simulink model "AEB_MODEL_F"  (R2022b)
settings: Solver=VariableStepAuto  StartTime=0.0  StopTime=10.0  RelTol=1e-3
model workspace (MAT data in the model file):
  DISTANCE = 100
  MASS_OF_THE_VEHICLE = 1500
  MIN_THRESHOLD_FOR_TTCmin = 0.7
  SPEED_OF_THE_EGO_VEHICLE = 80
  SPEED_OF_THE_LEADING_VEHICLE = 0
  TTC_EMERGE = 2
  Var = 0
libraries: simulink x37, spsOnDelayLib x1
(part 1 of 2)
Description:
  | VERSION 1.1
  | Done up to Brake pedal force calculation.
  | VERSION 1.2
  | Braking force applied from brake pedal force have been calculated.
  | VERSION 1.3
  | Calculating the required braking deceleration and setting the reaction time and following conditions.
  | VERSION 1.4
  | Both braking deceleration have been compared within the reaction time.
  | VERSION 1.5
  | logic gates are included to enable AEB system.
  | VERSION 1.6
  | Including some of the diagnostic check\fault and warning and condition for input range to enable AEB system through logic gate.
  | VERSION 1.7
  | Speed conversion kmph to m/s, distance to avoid collision have been calculated.
  | VERSION 1.8
  | Modelling condition for time phase partial braking.
  | VERSION 1.9
  | Modelled the condition for sudden action to apply full brake.
  | VERSION 1.10
  | Modelling the  for condition for TTCmin and TTCemerge.
  | VERSION 1.11
  | Modelling the minimum thershold for TTCmin and correcting the TTCemerge for full brake according to this TTCmin.
  | VERSION 1.12
  | Modelling the condition when to enable the full brake.
  | VERSION 1.13
  | modelled and checked the input for partial brake is correct when TTCmin have sufficient time.
  | VERSION 1.14
  | Modelling the partial brake in closed loop and limiting the braking decceleration with switch block.
  | VERSION 1.15
  | Correcting some errors by using switches and logic gates.
  | VERSION 1.16
  | Calculating the partial brake output is appropriate or not.
  | VERSION 1.17
  | Modelling the full brake in closed loop and limiting the braking decceleration with switch block.
  | VERSION 1.18
  | Recorrecting the errors occurred.
  | VERSION 1.19
  | Modelling the input condition for full brake and sudden action.
  | VERSION 1.20
  | Calculating the distance travelled after braking.
  | VERSION 1.21
  | Modelling the condition for AEB OFF at speed of ego and leading vehicle become equal.
  | VERSION 1.22
  | In output block switch is created to result the corresponding output finally.
  | VERSION 1.23
  | Indication were included for AEB status, partial brake, full brake, forward collision warning, manual mode, fault and warning.
  | VERSION 1.24
  | Updating the signal name, creating the subsystem for each calculations, proper routing line, proper naming.
  | VERSION 1.25
  | Removing the unwanted display.
  | VERSION 1.26
  | Correcting the error occurred. were the speed of ego and leading vehicle became zero AEB OFF at partial brake itself; while system is at full brake, so logic gate and switch block is included to overcome this error.
settings Model: Creator=Lenovo  LastModifiedBy=Lenovo

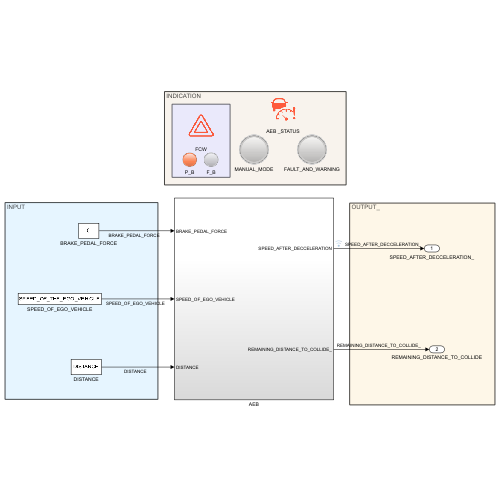
[thumbnail: Simulink's stored preview of the top-level diagram]
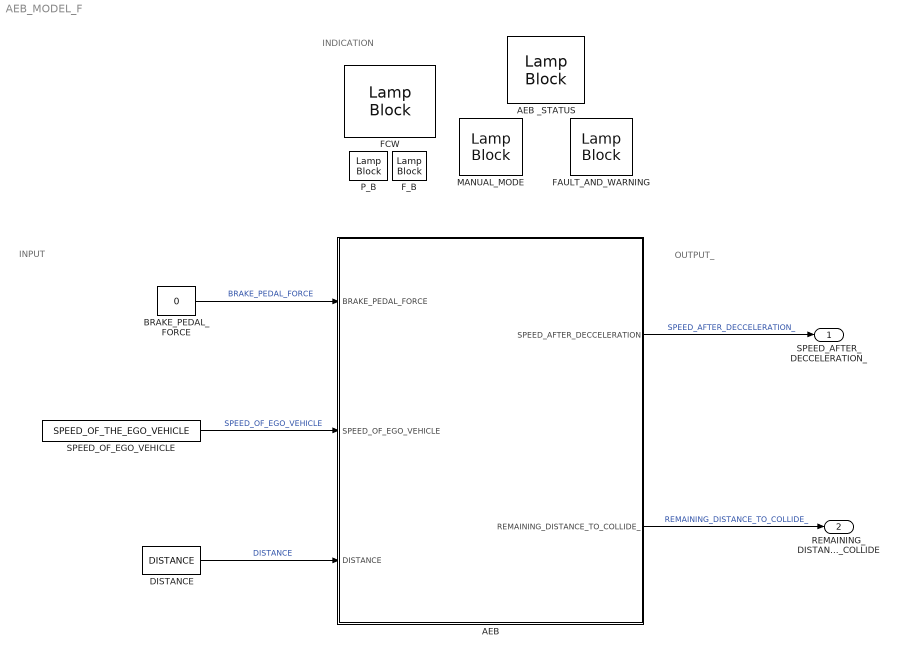
== system AEB_MODEL_F ==
  note: INPUT
  note: INDICATION
  note: OUTPUT_
  AEB : Subsystem
      settings: RTWMemSecFuncInitTerm=Inherit_from_model  RTWMemSecFuncExecute=Inherit_from_model  RTWMemSecDataConstants=Inherit_from_model  RTWMemSecDataInternal=Inherit_from_model  RTWMemSecDataParameters=Inherit_from_model
  AEB _STATUS : LampBlock  LabelPosition=Hide  Icon=AdaptiveCruiseControlFailure
  BRAKE_PEDAL_FORCE : Constant  Value=0
  DISTANCE : Constant  Value=DISTANCE
  FAULT_AND_WARNING : LampBlock  LabelPosition=Hide
  FCW : LampBlock  LabelPosition=Hide  Icon=Hazards
  F_B : LampBlock  LabelPosition=Hide
  MANUAL_MODE : LampBlock  LabelPosition=Hide
  P_B : LampBlock  LabelPosition=Hide
  SPEED_OF_EGO_VEHICLE : Constant  Value=SPEED_OF_THE_EGO_VEHICLE
  SPEED_AFTER_DECCELERATION_ : Outport
  REMAINING_DISTANCE_TO_COLLIDE : Outport  Port=2
  wires:
  AEB/2(REMAINING_DISTANCE_TO_COLLIDE_) -> REMAINING_DISTANCE_TO_COLLIDE/1  "REMAINING_DISTANCE_TO_COLLIDE_"
  DISTANCE/1 -> AEB/3(DISTANCE)  "DISTANCE"
  BRAKE_PEDAL_FORCE/1 -> AEB/1(BRAKE_PEDAL_FORCE)  "BRAKE_PEDAL_FORCE"
  AEB/1(SPEED_AFTER_DECCELERATION) -> SPEED_AFTER_DECCELERATION_/1  "SPEED_AFTER_DECCELERATION_"
  SPEED_OF_EGO_VEHICLE/1 -> AEB/2(SPEED_OF_EGO_VEHICLE)  "SPEED_OF_EGO_VEHICLE"

== system AEB_MODEL_F/AEB ==
  note: INPUT
  note: OUTPUT_
  BRAKE_PEDAL_FORCE : Inport
  SPEED_OF_EGO_VEHICLE : Inport  Port=2
  DISTANCE : Inport  Port=3
  AEB_SYSTEM : Subsystem
      settings: RTWMemSecFuncInitTerm=Inherit_from_model  RTWMemSecFuncExecute=Inherit_from_model  RTWMemSecDataConstants=Inherit_from_model  RTWMemSecDataInternal=Inherit_from_model  RTWMemSecDataParameters=Inherit_from_model
  BRAKE_PEDAL_FORCE_and_DIAGNOSTIC_CHECKS : Subsystem
      settings: RTWMemSecFuncInitTerm=Inherit_from_model  RTWMemSecFuncExecute=Inherit_from_model  RTWMemSecDataConstants=Inherit_from_model  RTWMemSecDataInternal=Inherit_from_model  RTWMemSecDataParameters=Inherit_from_model  PortSchema="{\"entries\":[{\"content\":{\"sides\":[{\"content\":{\"connectorIds\":[\"In1\",\"In2\",\"In3\"]},\"type\":\"ConnectorPlacement.EquallySpacedRectSide\",\"uuid\":\"3038f6ab-e2af-4165-8025-a57d9f66508d\"},{\"content\":{\"connectorIds\":[\"Out1\",\"Out2\"],\"side\":\"RIGHT\"},\"type\":\"ConnectorPlacement.EquallySpacedRectSide\",\"uuid\":\"1e43899d-0da6-488e-8e56-d64698be0fe8\"},{\"content\":{\"connectorIds\":[\"Out3\"],\"side\":\"TOP\"},\"type\":\"ConnectorPlacement.EquallySpacedRectSide\",\"uuid\":\"6462f150-b966-4129-881c-9cf441945b33\"}]},\"type\":\"ConnectorPlacement.EquallySpacedConnector\",\"uuid\":\"f400f814-be55-4fd0-9e8f-813a19493764\"}],\"packageUris\":[\"http://schema.mathworks.com/mf0/Connector/R2020b\"],\"version\":\"1.0\"}"
  SPEED_AFTER_DECCELERATION : Outport
  REMAINING_DISTANCE_TO_COLLIDE_ : Outport  Port=2
  wires:
  BRAKE_PEDAL_FORCE_and_DIAGNOSTIC_CHECKS/3(AEB_ENABLE) -> AEB_SYSTEM/Enable  "AEB_ENABLE"
  SPEED_OF_EGO_VEHICLE/1 -> BRAKE_PEDAL_FORCE_and_DIAGNOSTIC_CHECKS/2(SPEED_OF_EGO_VEHICLE)  "SPEED_OF_EGO_VEHICLE"
  BRAKE_PEDAL_FORCE/1 -> BRAKE_PEDAL_FORCE_and_DIAGNOSTIC_CHECKS/1(BRAKE_PEDAL_FORCE)  "BRAKE_PEDAL_FORCE"
  AEB_SYSTEM/1(SPEED_AFTER_DECCELERATION) -> SPEED_AFTER_DECCELERATION/1  "SPEED_AFTER_DECCELERATION"
  DISTANCE/1 -> BRAKE_PEDAL_FORCE_and_DIAGNOSTIC_CHECKS/3(DISTANCE)  "DISTANCE"
  AEB_SYSTEM/2(REMAINING_DISTANCE_TO_COLLIDE_) -> REMAINING_DISTANCE_TO_COLLIDE_/1  "REMAINING_DISTANCE_TO_COLLIDE"
  BRAKE_PEDAL_FORCE_and_DIAGNOSTIC_CHECKS/1(INITIAL_SPEED) -> AEB_SYSTEM/1(INITIAL_SPEED)  "INITIAL_SPEED"
  BRAKE_PEDAL_FORCE_and_DIAGNOSTIC_CHECKS/2(DISTANCE_TO_AVOID_COLLISION) -> AEB_SYSTEM/2(DISTANCE_TO_AVOID_COLLISION)  "DISTANCE_TO_AVOID_COLLISION"

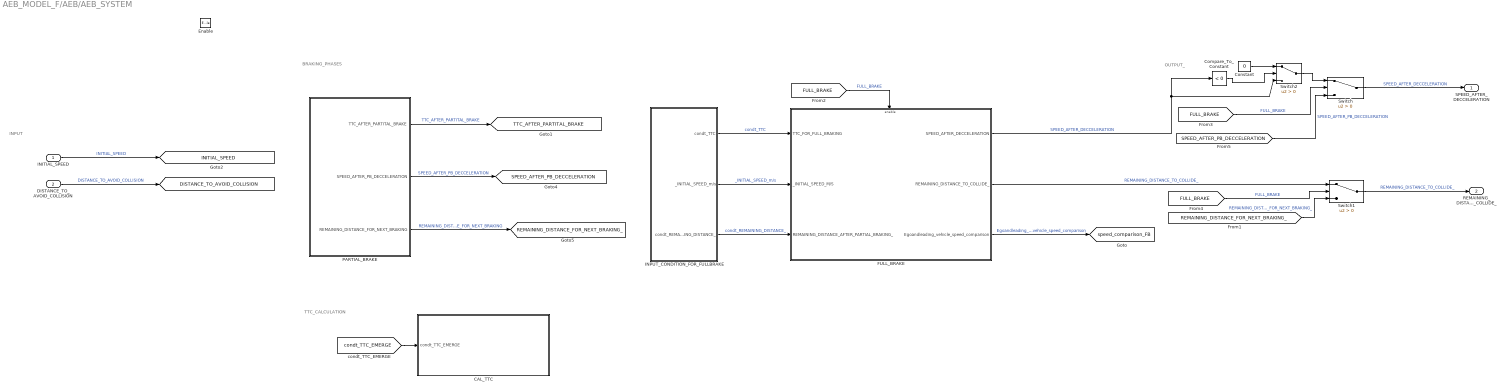
== system AEB_MODEL_F/AEB/AEB_SYSTEM ==
  note: OUTPUT_
  note: INPUT
  note: TTC_CALCULATION
  note: BRAKING_PHASES
  INITIAL_SPEED : Inport
  DISTANCE_TO_AVOID_COLLISION : Inport  Port=2
  Enable : EnablePort
  CAL_TTC : Subsystem
      settings: RTWMemSecFuncInitTerm=Inherit_from_model  RTWMemSecFuncExecute=Inherit_from_model  RTWMemSecDataConstants=Inherit_from_model  RTWMemSecDataInternal=Inherit_from_model  RTWMemSecDataParameters=Inherit_from_model
  Compare_To_Constant : simulink/Logic and Bit Operations/Compare To Constant  relop=<  const=0  OutDataTypeStr=boolean
      settings: RTWMemSecFuncInitTerm=Inherit_from_model  RTWMemSecFuncExecute=Inherit_from_model  RTWMemSecDataConstants=Inherit_from_model  RTWMemSecDataInternal=Inherit_from_model  RTWMemSecDataParameters=Inherit_from_model
  Constant : Constant  Value=0
  FULL_BRAKE : Subsystem
      settings: RTWMemSecFuncInitTerm=Inherit_from_model  RTWMemSecFuncExecute=Inherit_from_model  RTWMemSecDataConstants=Inherit_from_model  RTWMemSecDataInternal=Inherit_from_model  RTWMemSecDataParameters=Inherit_from_model
  INPUT_CONDITION_FOR_FULLBRAKE : Subsystem
      settings: RTWMemSecFuncInitTerm=Inherit_from_model  RTWMemSecFuncExecute=Inherit_from_model  RTWMemSecDataConstants=Inherit_from_model  RTWMemSecDataInternal=Inherit_from_model  RTWMemSecDataParameters=Inherit_from_model
  PARTIAL_BRAKE : Subsystem
      settings: RTWMemSecFuncInitTerm=Inherit_from_model  RTWMemSecFuncExecute=Inherit_from_model  RTWMemSecDataConstants=Inherit_from_model  RTWMemSecDataInternal=Inherit_from_model  RTWMemSecDataParameters=Inherit_from_model
  Switch : Switch  Criteria=u2 > Threshold  SaturateOnIntegerOverflow=off  InputSameDT=off
  Switch1 : Switch  Criteria=u2 > Threshold  SaturateOnIntegerOverflow=off  InputSameDT=off
  Switch2 : Switch  Criteria=u2 > Threshold  SaturateOnIntegerOverflow=off  InputSameDT=off
  SPEED_AFTER_DECCELERATION : Outport
  REMAINING_DISTANCE_TO_COLLIDE_ : Outport  Port=2
  tag scope: DISTANCE_TO_AVOID_COLLISION=global, INITIAL_SPEED=global, REMAINING_DISTANCE_FOR_NEXT_BRAKING_=global, SPEED_AFTER_PB_DECCELERATION=global, TTC_AFTER_PARTITAL_BRAKE=global, speed_comparison_FB=global
  wires:
  [condt_TTC_EMERGE] -> CAL_TTC/1(condt_TTC_EMERGE)
  [FULL_BRAKE] -> FULL_BRAKE/Enable  "FULL_BRAKE"
  PARTIAL_BRAKE/3(REMAINING_DISTANCE_FOR_NEXT_BRAKING) -> [REMAINING_DISTANCE_FOR_NEXT_BRAKING_]  "REMAINING_DISTANCE_FOR_NEXT_BRAKING"
  PARTIAL_BRAKE/2(SPEED_AFTER_PB_DECCELERATION) -> [SPEED_AFTER_PB_DECCELERATION]  "SPEED_AFTER_PB_DECCELERATION"
  PARTIAL_BRAKE/1(TTC_AFTER_PARTITAL_BRAKE) -> [TTC_AFTER_PARTITAL_BRAKE]  "TTC_AFTER_PARTITAL_BRAKE"
  INPUT_CONDITION_FOR_FULLBRAKE/1(condt_TTC) -> FULL_BRAKE/1(TTC_FOR_FULL_BRAKING)  "condt_TTC"
  INPUT_CONDITION_FOR_FULLBRAKE/2(_INITIAL_SPEED_m/s) -> FULL_BRAKE/2(_INITIAL_SPEED_M/S)  "_INITIAL_SPEED_m/s"
  INPUT_CONDITION_FOR_FULLBRAKE/3(condt_REMAINING_DISTANCE_) -> FULL_BRAKE/3(REMAINING_DISTANCE_AFTER_PARTIAL_BRAKING_)  "condt_REMAINING_DISTANCE_"
  Switch/1 -> SPEED_AFTER_DECCELERATION/1  "SPEED_AFTER_DECCELERATION"
  Switch1/1 -> REMAINING_DISTANCE_TO_COLLIDE_/1  "REMAINING_DISTANCE_TO_COLLIDE_"
  [REMAINING_DISTANCE_FOR_NEXT_BRAKING_] -> Switch1/3  "REMAINING_DISTANCE_FOR_NEXT_BRAKING_"
  [SPEED_AFTER_PB_DECCELERATION] -> Switch/3  "SPEED_AFTER_PB_DECCELERATION"
  [FULL_BRAKE] -> Switch/2  "FULL_BRAKE"
  [FULL_BRAKE] -> Switch1/2  "FULL_BRAKE"
  Compare_To_Constant/1 -> Switch2/2
  Constant/1 -> Switch2/1
  Switch2/1 -> Switch/1
  FULL_BRAKE/1(SPEED_AFTER_DECCELERATION) -> Compare_To_Constant/1, Switch2/3  "SPEED_AFTER_DECCELERATION"
  FULL_BRAKE/2(REMAINING_DISTANCE_TO_COLLIDE_) -> Switch1/1  "REMAINING_DISTANCE_TO_COLLIDE_"
  FULL_BRAKE/3(Egoandleading_vehicle_speed_comparison) -> [speed_comparison_FB]  "Egoandleading_vehicle_speed_comparison"
  INITIAL_SPEED/1 -> [INITIAL_SPEED]  "INITIAL_SPEED"
  DISTANCE_TO_AVOID_COLLISION/1 -> [DISTANCE_TO_AVOID_COLLISION]  "DISTANCE_TO_AVOID_COLLISION"

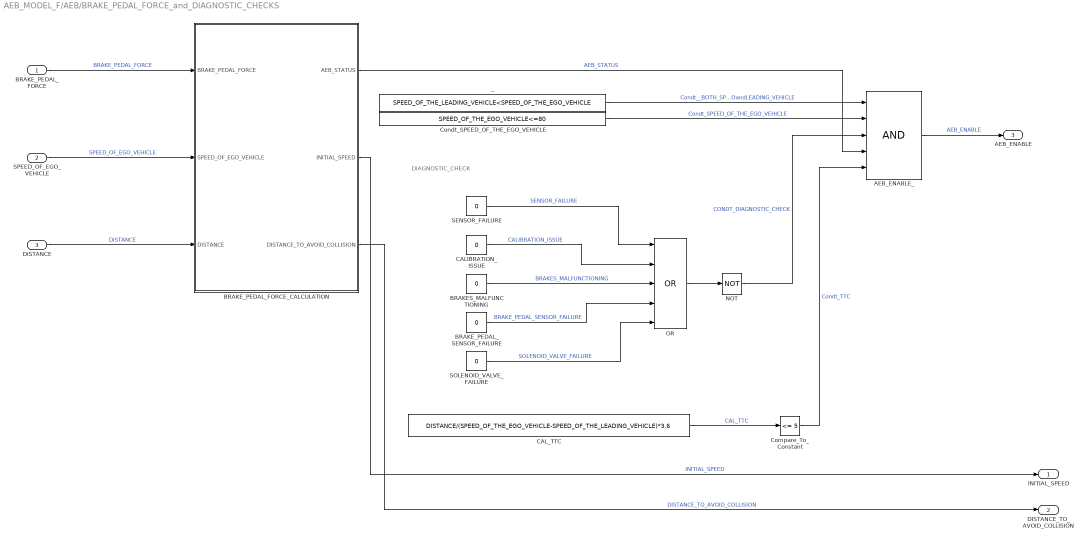
== system AEB_MODEL_F/AEB/BRAKE_PEDAL_FORCE_and_DIAGNOSTIC_CHECKS ==
  note: DIAGNOSTIC_CHECK
  BRAKE_PEDAL_FORCE : Inport
  SPEED_OF_EGO_VEHICLE : Inport  Port=2
  DISTANCE : Inport  Port=3
  AEB_ENABLE_ : Logic  Inputs=5  IconShape=distinctive  AllPortsSameDT=off  OutDataTypeStr=boolean
  BRAKES_MALFUNCTIONING : Constant  Value=0
  BRAKE_PEDAL_FORCE_CALCULATION : Subsystem
      settings: RTWMemSecFuncInitTerm=Inherit_from_model  RTWMemSecFuncExecute=Inherit_from_model  RTWMemSecDataConstants=Inherit_from_model  RTWMemSecDataInternal=Inherit_from_model  RTWMemSecDataParameters=Inherit_from_model
  BRAKE_PEDAL_SENSOR_FAILURE : Constant  Value=0
  CALIBRATION_ISSUE : Constant  Value=0
  CAL_TTC : Constant  Value=DISTANCE/(SPEED_OF_THE_EGO_VEHICLE-SPEED_OF_THE_LEADING_VEHICLE)*3.6
  Compare_To_Constant : simulink/Logic and Bit Operations/Compare To Constant  relop=<=  const=5  OutDataTypeStr=boolean
      settings: RTWMemSecFuncInitTerm=Inherit_from_model  RTWMemSecFuncExecute=Inherit_from_model  RTWMemSecDataConstants=Inherit_from_model  RTWMemSecDataInternal=Inherit_from_model  RTWMemSecDataParameters=Inherit_from_model
  Condt_SPEED_OF_THE_EGO_VEHICLE : Constant  Value=SPEED_OF_THE_EGO_VEHICLE<=80
  NOT : Logic  Operator=NOT  IconShape=distinctive  AllPortsSameDT=off  OutDataTypeStr=boolean
  OR : Logic  Operator=OR  Inputs=5  IconShape=distinctive  AllPortsSameDT=off  OutDataTypeStr=boolean
  SENSOR_FAILURE : Constant  Value=0
  SOLENOID_VALVE_FAILURE : Constant  Value=0
  _ : Constant  Value=SPEED_OF_THE_LEADING_VEHICLE<SPEED_OF_THE_EGO_VEHICLE
  INITIAL_SPEED : Outport
  DISTANCE_TO_AVOID_COLLISION : Outport  Port=2
  AEB_ENABLE : Outport  Port=3
  wires:
  BRAKES_MALFUNCTIONING/1 -> OR/3  "BRAKES_MALFUNCTIONING"
  BRAKE_PEDAL_FORCE/1 -> BRAKE_PEDAL_FORCE_CALCULATION/1(BRAKE_PEDAL_FORCE)  "BRAKE_PEDAL_FORCE"
  AEB_ENABLE_/1 -> AEB_ENABLE/1  "AEB_ENABLE"
  BRAKE_PEDAL_FORCE_CALCULATION/1(AEB_STATUS) -> AEB_ENABLE_/4  "AEB_STATUS"
  SENSOR_FAILURE/1 -> OR/1  "SENSOR_FAILURE"
  OR/1 -> NOT/1
  NOT/1 -> AEB_ENABLE_/3  "CONDT_DIAGNOSTIC_CHECK"
  BRAKE_PEDAL_SENSOR_FAILURE/1 -> OR/4  "BRAKE_PEDAL_SENSOR_FAILURE"
  CALIBRATION_ISSUE/1 -> OR/2  "CALIBRATION_ISSUE"
  _/1 -> AEB_ENABLE_/1  "Condt__BOTH_SPEED_OF_THE_EGOandLEADING_VEHICLE"
  Condt_SPEED_OF_THE_EGO_VEHICLE/1 -> AEB_ENABLE_/2  "Condt_SPEED_OF_THE_EGO_VEHICLE"
  SOLENOID_VALVE_FAILURE/1 -> OR/5  "SOLENOID_VALVE_FAILURE"
  CAL_TTC/1 -> Compare_To_Constant/1  "CAL_TTC"
  Compare_To_Constant/1 -> AEB_ENABLE_/5  "Condt_TTC"
  DISTANCE/1 -> BRAKE_PEDAL_FORCE_CALCULATION/3(DISTANCE)  "DISTANCE"
  SPEED_OF_EGO_VEHICLE/1 -> BRAKE_PEDAL_FORCE_CALCULATION/2(SPEED_OF_EGO_VEHICLE)  "SPEED_OF_EGO_VEHICLE"
  BRAKE_PEDAL_FORCE_CALCULATION/2(INITIAL_SPEED) -> INITIAL_SPEED/1  "INITIAL_SPEED"
  BRAKE_PEDAL_FORCE_CALCULATION/3(DISTANCE_TO_AVOID_COLLISION) -> DISTANCE_TO_AVOID_COLLISION/1  "DISTANCE_TO_AVOID_COLLISION"

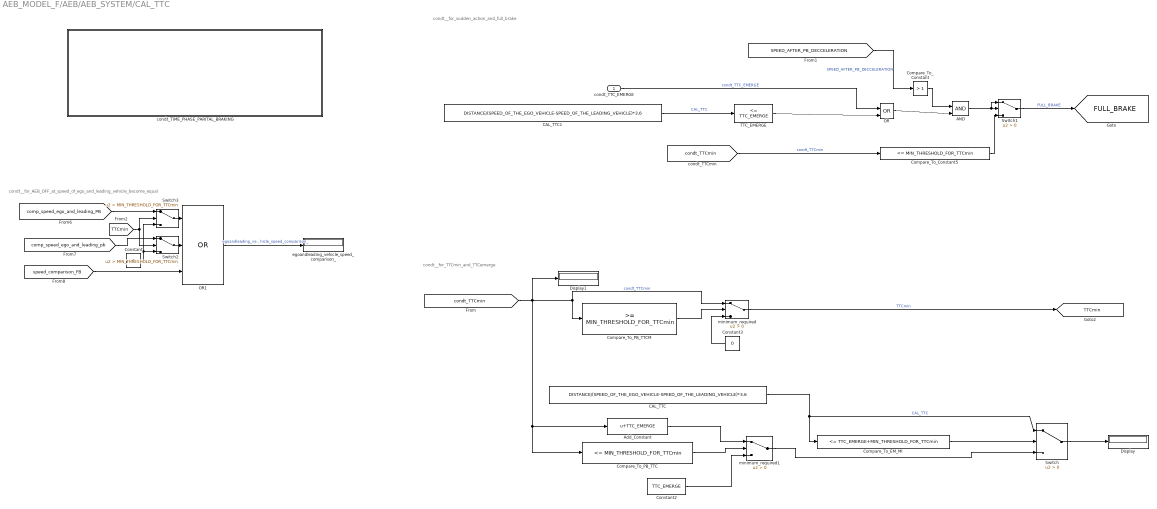
== system AEB_MODEL_F/AEB/AEB_SYSTEM/CAL_TTC ==
  note: condt__for_sudden_action_and_full_brake
  note: condt__for_TTCmin_and_TTCemerge
  note: condt__for_AEB_OFF_at_speed_of_ego_and_leading_vehicle_become_equal
  condt_TTC_EMERGE : Inport
  AND : Logic  IconShape=distinctive  AllPortsSameDT=off  OutDataTypeStr=boolean
  Add_Constant : Bias  Bias=TTC_EMERGE  SaturateOnIntegerOverflow=off
  CAL_TTC : Constant  Value=DISTANCE/(SPEED_OF_THE_EGO_VEHICLE-SPEED_OF_THE_LEADING_VEHICLE)*3.6
  CAL_TTC1 : Constant  Value=DISTANCE/(SPEED_OF_THE_EGO_VEHICLE-SPEED_OF_THE_LEADING_VEHICLE)*3.6
  Compare_To_Constant : simulink/Logic and Bit Operations/Compare To Constant  relop=>  const=1  OutDataTypeStr=boolean
      settings: RTWMemSecFuncInitTerm=Inherit_from_model  RTWMemSecFuncExecute=Inherit_from_model  RTWMemSecDataConstants=Inherit_from_model  RTWMemSecDataInternal=Inherit_from_model  RTWMemSecDataParameters=Inherit_from_model
  Compare_To_Constant5 : simulink/Logic and Bit Operations/Compare To Constant  relop=<=  const=MIN_THRESHOLD_FOR_TTCmin  OutDataTypeStr=boolean
      settings: RTWMemSecFuncInitTerm=Inherit_from_model  RTWMemSecFuncExecute=Inherit_from_model  RTWMemSecDataConstants=Inherit_from_model  RTWMemSecDataInternal=Inherit_from_model  RTWMemSecDataParameters=Inherit_from_model
  Compare_To_EM_MI : simulink/Logic and Bit Operations/Compare To Constant  relop=<=  const=TTC_EMERGE+MIN_THRESHOLD_FOR_TTCmin  OutDataTypeStr=boolean
      settings: RTWMemSecFuncInitTerm=Inherit_from_model  RTWMemSecFuncExecute=Inherit_from_model  RTWMemSecDataConstants=Inherit_from_model  RTWMemSecDataInternal=Inherit_from_model  RTWMemSecDataParameters=Inherit_from_model
  Compare_To_PB_TTC : simulink/Logic and Bit Operations/Compare To Constant  relop=<=  const=MIN_THRESHOLD_FOR_TTCmin  OutDataTypeStr=boolean
      settings: RTWMemSecFuncInitTerm=Inherit_from_model  RTWMemSecFuncExecute=Inherit_from_model  RTWMemSecDataConstants=Inherit_from_model  RTWMemSecDataInternal=Inherit_from_model  RTWMemSecDataParameters=Inherit_from_model
  Compare_To_PB_TTCM : simulink/Logic and Bit Operations/Compare To Constant  relop=>=  const=MIN_THRESHOLD_FOR_TTCmin  OutDataTypeStr=boolean
      settings: RTWMemSecFuncInitTerm=Inherit_from_model  RTWMemSecFuncExecute=Inherit_from_model  RTWMemSecDataConstants=Inherit_from_model  RTWMemSecDataInternal=Inherit_from_model  RTWMemSecDataParameters=Inherit_from_model
  Constant : Constant  Value=0
  Constant2 : Constant  Value=TTC_EMERGE
  Constant3 : Constant  Value=0
  Display : Display
  Display1 : Display
  OR : Logic  Operator=OR  IconShape=distinctive  AllPortsSameDT=off  OutDataTypeStr=boolean
  OR1 : Logic  Operator=OR  Inputs=3  IconShape=distinctive  AllPortsSameDT=off  OutDataTypeStr=boolean
  Switch : Switch  Criteria=u2 > Threshold  SaturateOnIntegerOverflow=off  InputSameDT=off
  Switch1 : Switch  Criteria=u2 > Threshold  SaturateOnIntegerOverflow=off  InputSameDT=off
  Switch2 : Switch  Criteria=u2 > Threshold  Threshold=MIN_THRESHOLD_FOR_TTCmin  SaturateOnIntegerOverflow=off  InputSameDT=off
  Switch3 : Switch  Criteria=u2 > Threshold  Threshold=MIN_THRESHOLD_FOR_TTCmin  SaturateOnIntegerOverflow=off  InputSameDT=off
  TTC_EMERGE : simulink/Logic and Bit Operations/Compare To Constant  relop=<=  const=TTC_EMERGE  OutDataTypeStr=boolean
      settings: RTWMemSecFuncInitTerm=Inherit_from_model  RTWMemSecFuncExecute=Inherit_from_model  RTWMemSecDataConstants=Inherit_from_model  RTWMemSecDataInternal=Inherit_from_model  RTWMemSecDataParameters=Inherit_from_model
  condt_TIME_PHASE_PARITAL_BRAKING : Subsystem
      settings: RTWMemSecFuncInitTerm=Inherit_from_model  RTWMemSecFuncExecute=Inherit_from_model  RTWMemSecDataConstants=Inherit_from_model  RTWMemSecDataInternal=Inherit_from_model  RTWMemSecDataParameters=Inherit_from_model
  egoandleading_vehicle_speed_comparison_ : Display
  minimum_required : Switch  Criteria=u2 > Threshold  SaturateOnIntegerOverflow=off  InputSameDT=off
  minimum_required1 : Switch  Criteria=u2 > Threshold  SaturateOnIntegerOverflow=off  InputSameDT=off
  tag scope: FULL_BRAKE=global, TTCmin=global
  wires:
  CAL_TTC1/1 -> TTC_EMERGE/1  "CAL_TTC"
  TTC_EMERGE/1 -> OR/2
  OR/1 -> AND/2
  condt_TTC_EMERGE/1 -> OR/1  "condt_TTC_EMERGE"
  [SPEED_AFTER_PB_DECCELERATION] -> Compare_To_Constant/1  "SPEED_AFTER_PB_DECCELERATION"
  Compare_To_Constant/1 -> AND/1
  AND/1 -> Switch1/1, Switch1/2
  Constant2/1 -> minimum_required1/3
  Constant3/1 -> minimum_required/3
  minimum_required/1 -> [TTCmin]  "TTCmin"
  [condt_TTCmin] -> Compare_To_PB_TTC/1, Add_Constant/1, Display1/1, minimum_required/1, Compare_To_PB_TTCM/1  "condt_TTCmin"
  Add_Constant/1 -> minimum_required1/1
  Compare_To_PB_TTCM/1 -> minimum_required/2
  minimum_required1/1 -> Switch/3
  Compare_To_PB_TTC/1 -> minimum_required1/2
  [condt_TTCmin] -> Compare_To_Constant5/1  "condt_TTCmin"
  Compare_To_Constant5/1 -> Switch1/3
  CAL_TTC/1 -> Compare_To_EM_MI/1, Switch/1  "CAL_TTC"
  Compare_To_EM_MI/1 -> Switch/2
  Switch1/1 -> [FULL_BRAKE]  "FULL_BRAKE"
  OR1/1 -> egoandleading_vehicle_speed_comparison_/1  "egoandleading_vehicle_speed_comparison_"
  [speed_comparison_FB] -> OR1/3
  [comp_speed_ego_and_leading_PB] -> Switch3/1
  [comp_speed_ego_and_leading_pb] -> Switch2/1
  Switch/1 -> Display/1
  Constant/1 -> Switch3/3, Switch2/3
  [TTCmin] -> Switch2/2, Switch3/2
  Switch2/1 -> OR1/2
  Switch3/1 -> OR1/1

== system AEB_MODEL_F/AEB/AEB_SYSTEM/FULL_BRAKE ==
  note: condt__for_AEB_OFF_at_speed_of_ego_and_leading_vehicle_become_equal
  note: OUTPUT
  note: INPUT
  TTC_FOR_FULL_BRAKING : Inport
  _INITIAL_SPEED_M/S : Inport  Port=2
  REMAINING_DISTANCE_AFTER_PARTIAL_BRAKING_ : Inport  Port=3
  Enable : EnablePort
  FB_CALCULATIONS : Subsystem
      settings: RTWMemSecFuncInitTerm=Inherit_from_model  RTWMemSecFuncExecute=Inherit_from_model  RTWMemSecDataConstants=Inherit_from_model  RTWMemSecDataInternal=Inherit_from_model  RTWMemSecDataParameters=Inherit_from_model
  FB_SYSTEM_IN_LOOP : Subsystem
      settings: RTWMemSecFuncInitTerm=Inherit_from_model  RTWMemSecFuncExecute=Inherit_from_model  RTWMemSecDataConstants=Inherit_from_model  RTWMemSecDataInternal=Inherit_from_model  RTWMemSecDataParameters=Inherit_from_model
  OR1 : Logic  Operator=OR  IconShape=distinctive  AllPortsSameDT=off  OutDataTypeStr=boolean
  SPEED_AFTER_DECCELERATION : Outport
  REMAINING_DISTANCE_TO_COLLIDE_ : Outport  Port=2
  Egoandleading_vehicle_speed_comparison : Outport  Port=3
  wires:
  FB_CALCULATIONS/1(TTC_FOR NEXT_BRAKE) -> FB_SYSTEM_IN_LOOP/1(TTC_AFTER_FULL_BRAKE)  "TTC_FOR NEXT_BRAKE"
  TTC_FOR_FULL_BRAKING/1 -> FB_CALCULATIONS/1(TTC_FOR_FULL_BRAKING)  "TTC_FOR_FULL_BRAKING"
  _INITIAL_SPEED_M/S/1 -> FB_CALCULATIONS/2(INITIAL_SPEED)  "_INITIAL_SPEED_M/S"
  FB_CALCULATIONS/2(SPEED_AFTER_FB_DECCELERATION) -> FB_SYSTEM_IN_LOOP/2(SPEED_AFTER_FB_DECCELERATION)  "SPEED_AFTER_FB_DECCELERATION"
  REMAINING_DISTANCE_AFTER_PARTIAL_BRAKING_/1 -> FB_CALCULATIONS/3(REMAINING_DISTANCE_AFTER_PARTIAL_BRAKING)  "REMAINING_DISTANCE_AFTER_PARTIAL_BRAKING_"
  OR1/1 -> Egoandleading_vehicle_speed_comparison/1
  [comp_speed_ego_and_leading2] -> OR1/1
  [comp_speed_ego_and_leading3] -> OR1/2
  FB_CALCULATIONS/3(REMAINING_DISTANCE_FOR_NEXT_BRAKING_) -> FB_SYSTEM_IN_LOOP/3(REMAINING_DISTANCE_FOR_NEXT_BRAKING_)  "REMAINING_DISTANCE_FOR_NEXT_BRAKING_"
  FB_SYSTEM_IN_LOOP/1(RATE_OF_SPEED) -> SPEED_AFTER_DECCELERATION/1  "SPEED_AFTER_DECCELERATION"
  FB_SYSTEM_IN_LOOP/2(RATE_OF_REMAINING_DISTANCE_FOR_NEXT_BRAKING_) -> REMAINING_DISTANCE_TO_COLLIDE_/1  "REMAINING_DISTANCE_TO_COLLIDE_"

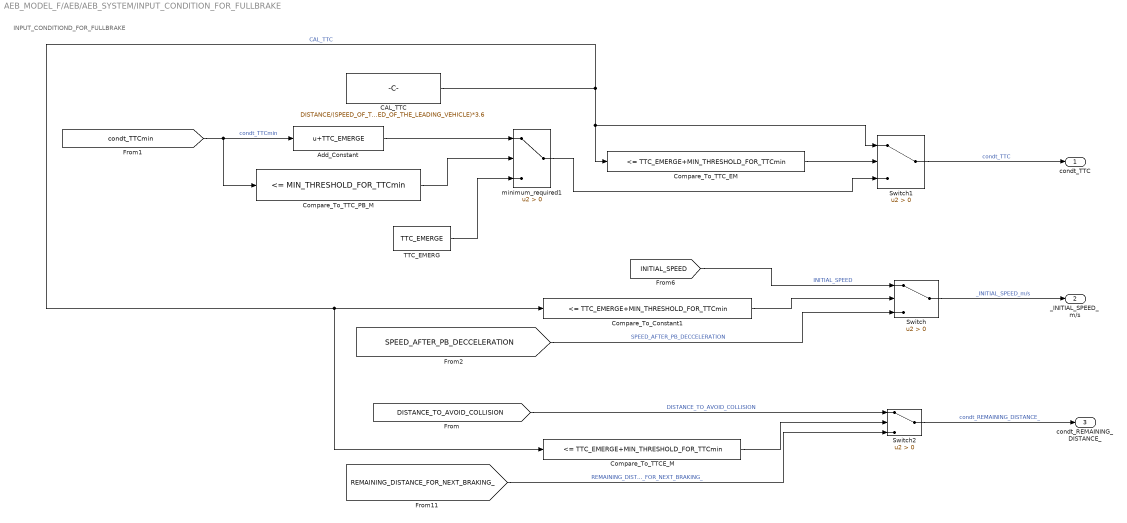
== system AEB_MODEL_F/AEB/AEB_SYSTEM/INPUT_CONDITION_FOR_FULLBRAKE ==
  note: INPUT_CONDITIOND_FOR_FULLBRAKE
  Add_Constant : Bias  Bias=TTC_EMERGE  SaturateOnIntegerOverflow=off
  CAL_TTC : Constant  Value=DISTANCE/(SPEED_OF_THE_EGO_VEHICLE-SPEED_OF_THE_LEADING_VEHICLE)*3.6
  Compare_To_Constant1 : simulink/Logic and Bit Operations/Compare To Constant  relop=<=  const=TTC_EMERGE+MIN_THRESHOLD_FOR_TTCmin  OutDataTypeStr=boolean
      settings: RTWMemSecFuncInitTerm=Inherit_from_model  RTWMemSecFuncExecute=Inherit_from_model  RTWMemSecDataConstants=Inherit_from_model  RTWMemSecDataInternal=Inherit_from_model  RTWMemSecDataParameters=Inherit_from_model
  Compare_To_TTCE_M : simulink/Logic and Bit Operations/Compare To Constant  relop=<=  const=TTC_EMERGE+MIN_THRESHOLD_FOR_TTCmin  OutDataTypeStr=boolean
      settings: RTWMemSecFuncInitTerm=Inherit_from_model  RTWMemSecFuncExecute=Inherit_from_model  RTWMemSecDataConstants=Inherit_from_model  RTWMemSecDataInternal=Inherit_from_model  RTWMemSecDataParameters=Inherit_from_model
  Compare_To_TTC_EM : simulink/Logic and Bit Operations/Compare To Constant  relop=<=  const=TTC_EMERGE+MIN_THRESHOLD_FOR_TTCmin  OutDataTypeStr=boolean
      settings: RTWMemSecFuncInitTerm=Inherit_from_model  RTWMemSecFuncExecute=Inherit_from_model  RTWMemSecDataConstants=Inherit_from_model  RTWMemSecDataInternal=Inherit_from_model  RTWMemSecDataParameters=Inherit_from_model
  Compare_To_TTC_PB_M : simulink/Logic and Bit Operations/Compare To Constant  relop=<=  const=MIN_THRESHOLD_FOR_TTCmin  OutDataTypeStr=boolean
      settings: RTWMemSecFuncInitTerm=Inherit_from_model  RTWMemSecFuncExecute=Inherit_from_model  RTWMemSecDataConstants=Inherit_from_model  RTWMemSecDataInternal=Inherit_from_model  RTWMemSecDataParameters=Inherit_from_model
  Switch : Switch  Criteria=u2 > Threshold  SaturateOnIntegerOverflow=off  InputSameDT=off
  Switch1 : Switch  Criteria=u2 > Threshold  SaturateOnIntegerOverflow=off  InputSameDT=off
  Switch2 : Switch  Criteria=u2 > Threshold  SaturateOnIntegerOverflow=off  InputSameDT=off
  TTC_EMERG : Constant  Value=TTC_EMERGE
  minimum_required1 : Switch  Criteria=u2 > Threshold  SaturateOnIntegerOverflow=off  InputSameDT=off
  condt_TTC : Outport
  _INITIAL_SPEED_m/s : Outport  Port=2
  condt_REMAINING_DISTANCE_ : Outport  Port=3
  wires:
  Switch/1 -> _INITIAL_SPEED_m/s/1  "_INITIAL_SPEED_m/s"
  [INITIAL_SPEED] -> Switch/1  "INITIAL_SPEED"
  Compare_To_Constant1/1 -> Switch/2
  Switch2/1 -> condt_REMAINING_DISTANCE_/1  "condt_REMAINING_DISTANCE_"
  Compare_To_TTCE_M/1 -> Switch2/2
  [REMAINING_DISTANCE_FOR_NEXT_BRAKING_] -> Switch2/3  "REMAINING_DISTANCE_FOR_NEXT_BRAKING_"
  [SPEED_AFTER_PB_DECCELERATION] -> Switch/3  "SPEED_AFTER_PB_DECCELERATION"
  [DISTANCE_TO_AVOID_COLLISION] -> Switch2/1  "DISTANCE_TO_AVOID_COLLISION"
  Switch1/1 -> condt_TTC/1  "condt_TTC"
  Add_Constant/1 -> minimum_required1/1
  CAL_TTC/1 -> Compare_To_TTC_EM/1, Switch1/1, Compare_To_Constant1/1, Compare_To_TTCE_M/1  "CAL_TTC"
  [condt_TTCmin] -> Compare_To_TTC_PB_M/1, Add_Constant/1  "condt_TTCmin"
  Compare_To_TTC_EM/1 -> Switch1/2
  TTC_EMERG/1 -> minimum_required1/3
  Compare_To_TTC_PB_M/1 -> minimum_required1/2
  minimum_required1/1 -> Switch1/3

== system AEB_MODEL_F/AEB/AEB_SYSTEM/PARTIAL_BRAKE ==
  note: PARTIAL_BRAKING
  note: OUTPUT_
  note: INPUT
  Constant : Constant  Value=0
  PARTIAL_BRAKING : Subsystem
      settings: RTWMemSecFuncInitTerm=Inherit_from_model  RTWMemSecFuncExecute=Inherit_from_model  RTWMemSecDataConstants=Inherit_from_model  RTWMemSecDataInternal=Inherit_from_model  RTWMemSecDataParameters=Inherit_from_model
  Switch : Switch  Criteria=u2 > Threshold  Threshold=MIN_THRESHOLD_FOR_TTCmin  SaturateOnIntegerOverflow=off  InputSameDT=off
  Switch2 : Switch  Criteria=u2 > Threshold  Threshold=MIN_THRESHOLD_FOR_TTCmin  SaturateOnIntegerOverflow=off  InputSameDT=off
  condt___TTC_EMERGE : simulink/Logic and Bit Operations/Compare To Constant  relop===  const=0  OutDataTypeStr=boolean
      settings: RTWMemSecFuncInitTerm=Inherit_from_model  RTWMemSecFuncExecute=Inherit_from_model  RTWMemSecDataConstants=Inherit_from_model  RTWMemSecDataInternal=Inherit_from_model  RTWMemSecDataParameters=Inherit_from_model
  TTC_AFTER_PARTITAL_BRAKE : Outport
  SPEED_AFTER_PB_DECCELERATION : Outport  Port=2
  REMAINING_DISTANCE_FOR_NEXT_BRAKING : Outport  Port=3
  tag scope: condt_TTC_EMERGE=global
  wires:
  condt___TTC_EMERGE/1 -> [condt_TTC_EMERGE]  "condt___TTC_EMERGE"
  PARTIAL_BRAKING/1(TTC_AFTER_PARTITAL_BRAKE) -> TTC_AFTER_PARTITAL_BRAKE/1, condt___TTC_EMERGE/1  "TTC_AFTER_PARTITAL_BRAKE"
  PARTIAL_BRAKING/3(REMAINING_DISTANCE_FOR_NEXT_BRAKING) -> REMAINING_DISTANCE_FOR_NEXT_BRAKING/1  "REMAINING_DISTANCE_FOR_NEXT_BRAKING"
  PARTIAL_BRAKING/2(SPEED_AFTER_PB_DECCELERATION) -> SPEED_AFTER_PB_DECCELERATION/1  "SPEED_AFTER_PB_DECCELERATION"
  Switch/1 -> PARTIAL_BRAKING/2(INITIAL_SPEED)  "INITIAL_SPEED"
  [INITIAL_SPEED] -> Switch/1
  Constant/1 -> Switch2/3, Switch/3
  [TTCmin] -> Switch/2, PARTIAL_BRAKING/3(TTCmin), Switch2/2  "TTCmin"
  Switch2/1 -> PARTIAL_BRAKING/1(DISTANCE_TO_AVOID_COLLISION)  "DISTANCE_TO_AVOID_COLLISION"
  [DISTANCE_TO_AVOID_COLLISION] -> Switch2/1

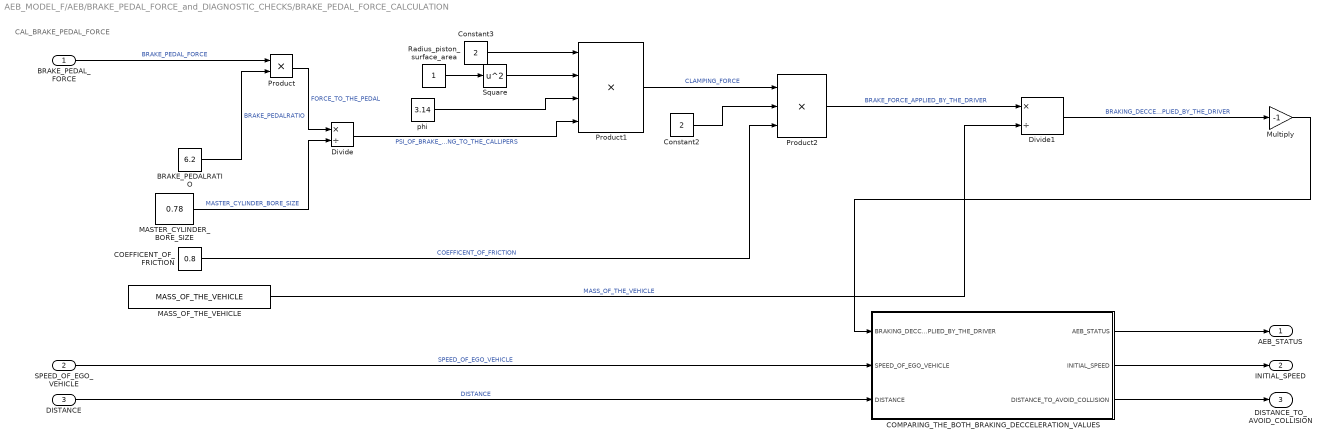
== system AEB_MODEL_F/AEB/BRAKE_PEDAL_FORCE_and_DIAGNOSTIC_CHECKS/BRAKE_PEDAL_FORCE_CALCULATION ==
  note: CAL_BRAKE_PEDAL_FORCE
  BRAKE_PEDAL_FORCE : Inport
  SPEED_OF_EGO_VEHICLE : Inport  Port=2
  DISTANCE : Inport  Port=3
  BRAKE_PEDALRATIO : Constant  Value=6.2
  COEFFICENT_OF_FRICTION : Constant  Value=0.8
  COMPARING_THE_BOTH_BRAKING_DECCELERATION_VALUES : Subsystem
      settings: RTWMemSecFuncInitTerm=Inherit_from_model  RTWMemSecFuncExecute=Inherit_from_model  RTWMemSecDataConstants=Inherit_from_model  RTWMemSecDataInternal=Inherit_from_model  RTWMemSecDataParameters=Inherit_from_model
  Constant2 : Constant  Value=2
  Constant3 : Constant  Value=2
  Divide : Product  Inputs=*/
  Divide1 : Product  Inputs=*/
  MASS_OF_THE_VEHICLE : Constant  Value=MASS_OF_THE_VEHICLE
  MASTER_CYLINDER_BORE_SIZE : Constant  Value=0.78
  Multiply : Gain  Gain=-1
  Product : Product
  Product1 : Product  Inputs=4
  Product2 : Product  Inputs=3
  Radius_piston_surface_area : Constant
  Square : Math  Operator=square
  phi : Constant  Value=3.14
  AEB_STATUS : Outport
  INITIAL_SPEED : Outport  Port=2
  DISTANCE_TO_AVOID_COLLISION : Outport  Port=3
  wires:
  Product2/1 -> Divide1/1  "BRAKE_FORCE_APPLIED_BY_THE_DRIVER"
  Product/1 -> Divide/1  "FORCE_TO_THE_PEDAL"
  COEFFICENT_OF_FRICTION/1 -> Product2/3  "COEFFICENT_OF_FRICTION"
  Divide/1 -> Product1/4  "PSI_OF_BRAKE_FULID_HEADING_TO_THE_CALLIPERS"
  BRAKE_PEDALRATIO/1 -> Product/2  "BRAKE_PEDALRATIO"
  phi/1 -> Product1/3
  BRAKE_PEDAL_FORCE/1 -> Product/1  "BRAKE_PEDAL_FORCE"
  MASS_OF_THE_VEHICLE/1 -> Divide1/2  "MASS_OF_THE_VEHICLE"
  Radius_piston_surface_area/1 -> Square/1
  Square/1 -> Product1/2
  Constant2/1 -> Product2/2
  MASTER_CYLINDER_BORE_SIZE/1 -> Divide/2  "MASTER_CYLINDER_BORE_SIZE"
  Product1/1 -> Product2/1  "CLAMPING_FORCE"
  Constant3/1 -> Product1/1
  Divide1/1 -> Multiply/1  "BRAKING_DECCELERATION_APPLIED_BY_THE_DRIVER"
  COMPARING_THE_BOTH_BRAKING_DECCELERATION_VALUES/1(AEB_STATUS) -> AEB_STATUS/1
  Multiply/1 -> COMPARING_THE_BOTH_BRAKING_DECCELERATION_VALUES/1(BRAKING_DECCELERATION_APPLIED_BY_THE_DRIVER)
  SPEED_OF_EGO_VEHICLE/1 -> COMPARING_THE_BOTH_BRAKING_DECCELERATION_VALUES/2(SPEED_OF_EGO_VEHICLE)  "SPEED_OF_EGO_VEHICLE"
  DISTANCE/1 -> COMPARING_THE_BOTH_BRAKING_DECCELERATION_VALUES/3(DISTANCE)  "DISTANCE"
  COMPARING_THE_BOTH_BRAKING_DECCELERATION_VALUES/2(INITIAL_SPEED) -> INITIAL_SPEED/1
  COMPARING_THE_BOTH_BRAKING_DECCELERATION_VALUES/3(DISTANCE_TO_AVOID_COLLISION) -> DISTANCE_TO_AVOID_COLLISION/1

== system AEB_MODEL_F/AEB/AEB_SYSTEM/CAL_TTC/condt_TIME_PHASE_PARITAL_BRAKING ==
  CAL_TTC : Constant  Value=DISTANCE/(SPEED_OF_THE_EGO_VEHICLE-SPEED_OF_THE_LEADING_VEHICLE)*3.6
  Compare_To_Constant : simulink/Logic and Bit Operations/Compare To Constant  relop=>=  const=5  OutDataTypeStr=boolean
      settings: RTWMemSecFuncInitTerm=Inherit_from_model  RTWMemSecFuncExecute=Inherit_from_model  RTWMemSecDataConstants=Inherit_from_model  RTWMemSecDataInternal=Inherit_from_model  RTWMemSecDataParameters=Inherit_from_model
  Compare_To_Constant1 : simulink/Logic and Bit Operations/Compare To Constant  relop=<  const=0  OutDataTypeStr=boolean
      settings: RTWMemSecFuncInitTerm=Inherit_from_model  RTWMemSecFuncExecute=Inherit_from_model  RTWMemSecDataConstants=Inherit_from_model  RTWMemSecDataInternal=Inherit_from_model  RTWMemSecDataParameters=Inherit_from_model
  Constant : Constant  Value=0
  REACTION TIME : Constant
  REACTION_TIME : Subsystem
      settings: RTWMemSecFuncInitTerm=Inherit_from_model  RTWMemSecFuncExecute=Inherit_from_model  RTWMemSecDataConstants=Inherit_from_model  RTWMemSecDataInternal=Inherit_from_model  RTWMemSecDataParameters=Inherit_from_model
  Subtract2 : Sum  Inputs=+--
  Switch : Switch  Criteria=u2 > Threshold  SaturateOnIntegerOverflow=off  InputSameDT=off
  TTC_EMERGE : Constant  Value=TTC_EMERGE
  tag scope: condt_TTCmin=global
  wires:
  CAL_TTC/1 -> Compare_To_Constant/1, Subtract2/1  "CAL_TTC"
  TTC_EMERGE/1 -> Subtract2/3  "TTC_EMERGE"
  REACTION_TIME/1(Out1) -> Subtract2/2  "REACTION_TIME"
  REACTION TIME/1 -> REACTION_TIME/1(In1)  "REACTION TIME"
  Compare_To_Constant/1 -> REACTION_TIME/Enable
  Subtract2/1 -> Switch/3, Compare_To_Constant1/1  "TTC_PARITAL_BRAKING"
  Compare_To_Constant1/1 -> Switch/2
  Constant/1 -> Switch/1
  Switch/1 -> [condt_TTCmin]  "condt_TTCmin"

== system AEB_MODEL_F/AEB/AEB_SYSTEM/FULL_BRAKE/FB_CALCULATIONS ==
  note: ego_and_leading_vehicle_speed_comparison
  TTC_FOR_FULL_BRAKING : Inport
  INITIAL_SPEED : Inport  Port=2
  REMAINING_DISTANCE_AFTER_PARTIAL_BRAKING : Inport  Port=3
  CAL_BRAKING_DECCELERATION : Subsystem
      settings: RTWMemSecFuncInitTerm=Inherit_from_model  RTWMemSecFuncExecute=Inherit_from_model  RTWMemSecDataConstants=Inherit_from_model  RTWMemSecDataInternal=Inherit_from_model  RTWMemSecDataParameters=Inherit_from_model
  CAL_TTC : Subsystem
      settings: RTWMemSecFuncInitTerm=Inherit_from_model  RTWMemSecFuncExecute=Inherit_from_model  RTWMemSecDataConstants=Inherit_from_model  RTWMemSecDataInternal=Inherit_from_model  RTWMemSecDataParameters=Inherit_from_model
  CAL_inital_after_decceleration_speed : Subsystem
      settings: RTWMemSecFuncInitTerm=Inherit_from_model  RTWMemSecFuncExecute=Inherit_from_model  RTWMemSecDataConstants=Inherit_from_model  RTWMemSecDataInternal=Inherit_from_model  RTWMemSecDataParameters=Inherit_from_model
  CAL_remainig_distance : Subsystem
      settings: RTWMemSecFuncInitTerm=Inherit_from_model  RTWMemSecFuncExecute=Inherit_from_model  RTWMemSecDataConstants=Inherit_from_model  RTWMemSecDataInternal=Inherit_from_model  RTWMemSecDataParameters=Inherit_from_model
  Compare_To_Constant : simulink/Logic and Bit Operations/Compare To Constant  relop=<=  const=SPEED_OF_THE_LEADING_VEHICLE  OutDataTypeStr=boolean
      settings: RTWMemSecFuncInitTerm=Inherit_from_model  RTWMemSecFuncExecute=Inherit_from_model  RTWMemSecDataConstants=Inherit_from_model  RTWMemSecDataInternal=Inherit_from_model  RTWMemSecDataParameters=Inherit_from_model
  Constant : Constant  Value=0
  KM/hr to M/hr : Gain  Gain=3.6
  Switch : Switch  Criteria=u2 > Threshold  SaturateOnIntegerOverflow=off  InputSameDT=off
  TTC_FOR NEXT_BRAKE : Outport
  SPEED_AFTER_FB_DECCELERATION : Outport  Port=2
  REMAINING_DISTANCE_FOR_NEXT_BRAKING_ : Outport  Port=3
  tag scope: comp_speed_ego_and_leading2=global
  wires:
  CAL_BRAKING_DECCELERATION/1(FB_DECCELERATION) -> CAL_remainig_distance/4(FB_DECCELERATION), CAL_inital_after_decceleration_speed/3(FULL_BRAKING_DECCELERATION)  "FB_DECCELERATION"
  INITIAL_SPEED/1 -> CAL_remainig_distance/1(INITIAL_SPEED), CAL_inital_after_decceleration_speed/1(INITIAL_SPEED), CAL_BRAKING_DECCELERATION/2(INITIAL_SPEED)  "INITIAL_SPEED"
  TTC_FOR_FULL_BRAKING/1 -> CAL_inital_after_decceleration_speed/2(TTC_FOR_FULL_BRAKING), CAL_remainig_distance/3(TTC_FOR_FULL_BRAKING)  "TTC_FOR_FULL_BRAKING"
  CAL_inital_after_decceleration_speed/1(INITIAL_SPEED_M/S) -> CAL_TTC/1(INITIAL_SPEED_M/S)  "INITIAL_SPEED_M/S"
  REMAINING_DISTANCE_AFTER_PARTIAL_BRAKING/1 -> CAL_remainig_distance/2(REMAINING_DISTANCE_AFTER_PARTIAL_BRAKING), CAL_BRAKING_DECCELERATION/1(REMAINING_DISTANCE_AFTER_PARTIAL_BRAKING)  "REMAINING_DISTANCE_AFTER_PARTIAL_BRAKING"
  CAL_inital_after_decceleration_speed/2(SPEED_AFTER_FB_DECCELERATION) -> Switch/3, KM/hr to M/hr/1  "SPEED_AFTER_FB_DECCELERATION"
  CAL_TTC/1(TTC_FOR_FULL_BRAKING) -> TTC_FOR NEXT_BRAKE/1  "TTC_FOR NEXT_BRAKE"
  CAL_remainig_distance/1(remainig_distance) -> CAL_TTC/2(SPEED_AFTER_FB_DECCELERATION), REMAINING_DISTANCE_FOR_NEXT_BRAKING_/1  "REMAINING_DISTANCE_FOR_NEXT_BRAKING_"
  KM/hr to M/hr/1 -> Compare_To_Constant/1
  Compare_To_Constant/1 -> Switch/2, [comp_speed_ego_and_leading2]
  Constant/1 -> Switch/1
  Switch/1 -> SPEED_AFTER_FB_DECCELERATION/1

== system AEB_MODEL_F/AEB/AEB_SYSTEM/FULL_BRAKE/FB_SYSTEM_IN_LOOP ==
  note: condt_distance_travelled_after_brake
  TTC_AFTER_FULL_BRAKE : Inport
  SPEED_AFTER_FB_DECCELERATION : Inport  Port=2
  REMAINING_DISTANCE_FOR_NEXT_BRAKING_ : Inport  Port=3
  Add : Sum  Inputs=+-
  CALCULATIONS_WITH_RESPECT_TO_TTC : Subsystem
      settings: RTWMemSecFuncInitTerm=Inherit_from_model  RTWMemSecFuncExecute=Inherit_from_model  RTWMemSecDataConstants=Inherit_from_model  RTWMemSecDataInternal=Inherit_from_model  RTWMemSecDataParameters=Inherit_from_model
  Constant : Constant  Value=0
  Constant1 : Constant  Value=DISTANCE
  DISTANCE_TO_AVOID_COLLISION : Constant
  REMAINING_DISTANCE : Subsystem
      settings: RTWMemSecFuncInitTerm=Inherit_from_model  RTWMemSecFuncExecute=Inherit_from_model  RTWMemSecDataConstants=Inherit_from_model  RTWMemSecDataInternal=Inherit_from_model  RTWMemSecDataParameters=Inherit_from_model
  SPEED : Subsystem
      settings: RTWMemSecFuncInitTerm=Inherit_from_model  RTWMemSecFuncExecute=Inherit_from_model  RTWMemSecDataConstants=Inherit_from_model  RTWMemSecDataInternal=Inherit_from_model  RTWMemSecDataParameters=Inherit_from_model
  Subtract : Sum  Inputs=+-
  Switch : Switch  Criteria=u2 > Threshold  SaturateOnIntegerOverflow=off  InputSameDT=off
  TTC_AFTER_FULL_BRAKING : Subsystem
      settings: RTWMemSecFuncInitTerm=Inherit_from_model  RTWMemSecFuncExecute=Inherit_from_model  RTWMemSecDataConstants=Inherit_from_model  RTWMemSecDataInternal=Inherit_from_model  RTWMemSecDataParameters=Inherit_from_model
  RATE_OF_SPEED : Outport
  RATE_OF_REMAINING_DISTANCE_FOR_NEXT_BRAKING_ : Outport  Port=2
  wires:
  CALCULATIONS_WITH_RESPECT_TO_TTC/2(SPEED_AFTER_DECCELERATION) -> SPEED/2(NEXT_ITERATION)  "NEXT_ITERATION"
  REMAINING_DISTANCE/1(RATE_OF_REMAINING_DISTANCE_FOR_NEXT_BRAKING_) -> RATE_OF_REMAINING_DISTANCE_FOR_NEXT_BRAKING_/1, Switch/2, Subtract/2  "RATE_OF_REMAINING_DISTANCE_FOR_NEXT_BRAKING_"
  CALCULATIONS_WITH_RESPECT_TO_TTC/3(REMAINING_DISTANCE_FOR_NEXT_BRAKING_) -> REMAINING_DISTANCE/2(NEXT_ITERATION)  "NEXT_ITERATION"
  REMAINING_DISTANCE/2(CAL__REMAINING_DISTANCE_FOR_NEXT_BRAKING_) -> CALCULATIONS_WITH_RESPECT_TO_TTC/1(DISTANCE_TO_AVOID_COLLISION)  "CAL__REMAINING_DISTANCE_FOR_NEXT_BRAKING_"
  SPEED/2(CAL__SPEED_AFTER_DECCELERATION) -> CALCULATIONS_WITH_RESPECT_TO_TTC/2(INITIAL_SPEED)  "CAL__SPEED_AFTER_DECCELERATION"
  SPEED/1(RATE_OF _SPEED) -> RATE_OF_SPEED/1  "RATE_OF _SPEED"
  SPEED_AFTER_FB_DECCELERATION/1 -> SPEED/1(SPEED_AFTER_FB_DECCELERATION)  "SPEED_AFTER_FB_DECCELERATION"
  REMAINING_DISTANCE_FOR_NEXT_BRAKING_/1 -> REMAINING_DISTANCE/1(REMAINING_DISTANCE_FOR_NEXT_BRAKING_)  "REMAINING_DISTANCE_FOR_NEXT_BRAKING_"
  TTC_AFTER_FULL_BRAKING/2(CAL__TTC_FULL_BRAKE) -> CALCULATIONS_WITH_RESPECT_TO_TTC/3(TTC_FB_IN)  "CAL__TTC_FULL_BRAKE"
  CALCULATIONS_WITH_RESPECT_TO_TTC/1(TTC_AFTER_FULL_BRAKE) -> TTC_AFTER_FULL_BRAKING/2(NEXT_ITERATION)  "NEXT_ITERATION"
  TTC_AFTER_FULL_BRAKE/1 -> TTC_AFTER_FULL_BRAKING/1(TTC_AFTER_FULL_BRAKE)  "TTC_AFTER_FULL_BRAKE"
  Switch/1 -> ?  "distance_travelled_after_brake"
  Constant/1 -> Switch/3
  Subtract/1 -> Switch/1
  Add/1 -> Subtract/1
  Constant1/1 -> Add/1  "DISTANCE"
  DISTANCE_TO_AVOID_COLLISION/1 -> Add/2

== system AEB_MODEL_F/AEB/AEB_SYSTEM/PARTIAL_BRAKE/PARTIAL_BRAKING ==
  DISTANCE_TO_AVOID_COLLISION : Inport
  INITIAL_SPEED : Inport  Port=2
  TTCmin : Inport  Port=3
  PB_CALCULATIONS : Subsystem
      settings: RTWMemSecFuncInitTerm=Inherit_from_model  RTWMemSecFuncExecute=Inherit_from_model  RTWMemSecDataConstants=Inherit_from_model  RTWMemSecDataInternal=Inherit_from_model  RTWMemSecDataParameters=Inherit_from_model
  PB_IN_LOOP : Subsystem
      settings: RTWMemSecFuncInitTerm=Inherit_from_model  RTWMemSecFuncExecute=Inherit_from_model  RTWMemSecDataConstants=Inherit_from_model  RTWMemSecDataInternal=Inherit_from_model  RTWMemSecDataParameters=Inherit_from_model
  TTC_AFTER_PARTITAL_BRAKE : Outport
  SPEED_AFTER_PB_DECCELERATION : Outport  Port=2
  REMAINING_DISTANCE_FOR_NEXT_BRAKING : Outport  Port=3
  wires:
  INITIAL_SPEED/1 -> PB_CALCULATIONS/2(INITIAL_SPEED)  "INITIAL_SPEED"
  DISTANCE_TO_AVOID_COLLISION/1 -> PB_CALCULATIONS/1(DISTANCE_TO_AVOID_COLLISION)  "DISTANCE_TO_AVOID_COLLISION"
  PB_IN_LOOP/2(RATE_OF_SPEED) -> SPEED_AFTER_PB_DECCELERATION/1  "SPEED_AFTER_PB_DECCELERATION"
  TTCmin/1 -> PB_CALCULATIONS/3(TTCmin)  "TTCmin"
  PB_IN_LOOP/1(RATE_OF_ TTC_AFTER_PARTITAL_BRAKE) -> TTC_AFTER_PARTITAL_BRAKE/1  "TTC_AFTER_PARTITAL_BRAKE"
  PB_IN_LOOP/3(RATE_OF _REMAINING_DISTANCE_FOR_NEXT_BRAKING_) -> REMAINING_DISTANCE_FOR_NEXT_BRAKING/1  "REMAINING_DISTANCE_FOR_NEXT_BRAKING"
  PB_CALCULATIONS/1(TTC_AFTER_PARTITAL_BRAKE) -> PB_IN_LOOP/1(TTC_AFTER_PARTITAL_BRAKE)  "TTC_AFTER_PARTITAL_BRAKE"
  PB_CALCULATIONS/2(SPEED_AFTER_PB_DECCELERATION) -> PB_IN_LOOP/2(_SPEED_AFTER_PB_DECCELERATION)  "SPEED_AFTER_PB_DECCELERATION"
  PB_CALCULATIONS/3(REMAINING_DISTANCE_FOR_NEXT_BRAKING) -> PB_IN_LOOP/3(REMAINING_DISTANCE_FOR_NEXT_BRAKING_)  "REMAINING_DISTANCE_FOR_NEXT_BRAKING"

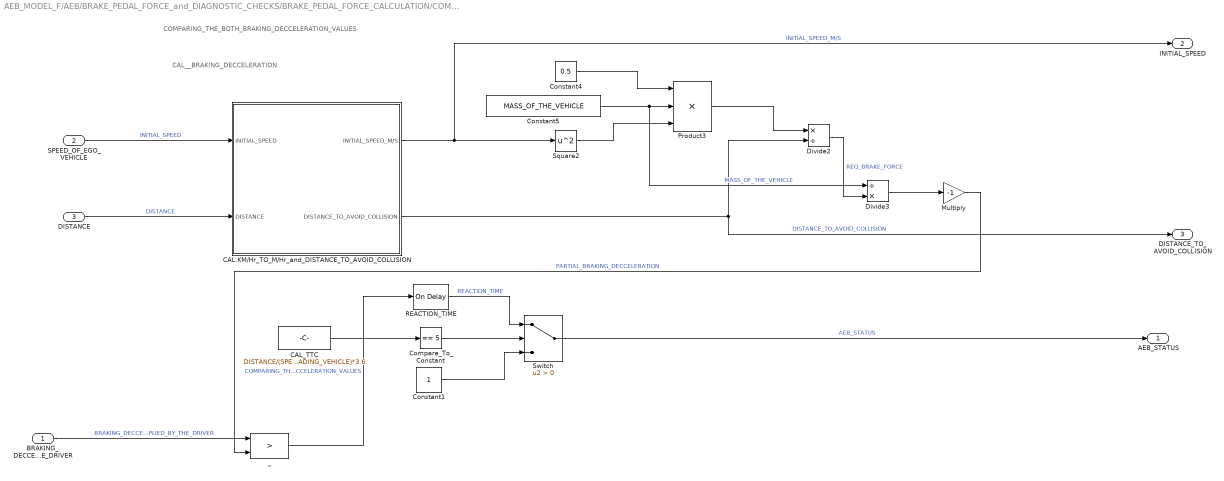
== system AEB_MODEL_F/AEB/BRAKE_PEDAL_FORCE_and_DIAGNOSTIC_CHECKS/BRAKE_PEDAL_FORCE_CALCULATION/COMPARING_THE_BOTH_BRAKING_DECCELERATION_VALUES ==
  note: COMPARING_THE_BOTH_BRAKING_DECCELERATION_VALUES
  note: CAL__BRAKING_DECCELERATION
  BRAKING_DECCELERATION_APPLIED_BY_THE_DRIVER : Inport
  SPEED_OF_EGO_VEHICLE : Inport  Port=2
  DISTANCE : Inport  Port=3
  CAL.KM/Hr_TO_M/Hr_and_DISTANCE_TO_AVOID_COLLISION : Subsystem
      settings: RTWMemSecFuncInitTerm=Inherit_from_model  RTWMemSecFuncExecute=Inherit_from_model  RTWMemSecDataConstants=Inherit_from_model  RTWMemSecDataInternal=Inherit_from_model  RTWMemSecDataParameters=Inherit_from_model
  CAL_TTC : Constant  Value=DISTANCE/(SPEED_OF_THE_EGO_VEHICLE-SPEED_OF_THE_LEADING_VEHICLE)*3.6
  Compare_To_Constant : simulink/Logic and Bit Operations/Compare To Constant  relop===  const=5  OutDataTypeStr=boolean
      settings: RTWMemSecFuncInitTerm=Inherit_from_model  RTWMemSecFuncExecute=Inherit_from_model  RTWMemSecDataConstants=Inherit_from_model  RTWMemSecDataInternal=Inherit_from_model  RTWMemSecDataParameters=Inherit_from_model
  Constant1 : Constant
  Constant4 : Constant  Value=0.5
  Constant5 : Constant  Value=MASS_OF_THE_VEHICLE
  Divide2 : Product  Inputs=*/
  Divide3 : Product  Inputs=/*
  Multiply : Gain  Gain=-1
  Product3 : Product  Inputs=3
  REACTION_TIME : spsOnDelayLib/On Delay  DelayType=On delay  delay=1  ic=0  Ts=0
      link override Model: ScheduleAs=Sample time
      link override Model/OFF Delay/Edge Detector/Model: ScheduleAs=Sample time
      link override Model/OFF Delay/Sample_and_Hold/Model: ScheduleAs=Sample time
      link override Model/ON Delay/Edge Detector/Model: ScheduleAs=Sample time
      link override Model/ON Delay/Sample_and_Hold/Model: ScheduleAs=Sample time
      settings: RTWMemSecFuncInitTerm=Inherit_from_model  RTWMemSecFuncExecute=Inherit_from_model  RTWMemSecDataConstants=Inherit_from_model  RTWMemSecDataInternal=Inherit_from_model  RTWMemSecDataParameters=Inherit_from_model
      link override Model: RTWMemSecFuncInitTerm=Inherit_from_model  RTWMemSecFuncExecute=Inherit_from_model  RTWMemSecDataConstants=Inherit_from_model  RTWMemSecDataInternal=Inherit_from_model  RTWMemSecDataParameters=Inherit_from_model
      link override Model/OFF Delay/Edge Detector/Model: RTWMemSecFuncInitTerm=Inherit_from_model  RTWMemSecFuncExecute=Inherit_from_model  RTWMemSecDataConstants=Inherit_from_model  RTWMemSecDataInternal=Inherit_from_model  RTWMemSecDataParameters=Inherit_from_model
      link override Model/OFF Delay/Edge_Detector: RTWMemSecFuncInitTerm=Inherit_from_model  RTWMemSecFuncExecute=Inherit_from_model  RTWMemSecDataConstants=Inherit_from_model  RTWMemSecDataInternal=Inherit_from_model  RTWMemSecDataParameters=Inherit_from_model
      link override Model/OFF Delay/Sample_and_Hold: RTWMemSecFuncInitTerm=Inherit_from_model  RTWMemSecFuncExecute=Inherit_from_model  RTWMemSecDataConstants=Inherit_from_model  RTWMemSecDataInternal=Inherit_from_model  RTWMemSecDataParameters=Inherit_from_model
      link override Model/OFF Delay/Sample_and_Hold/Model: RTWMemSecFuncInitTerm=Inherit_from_model  RTWMemSecFuncExecute=Inherit_from_model  RTWMemSecDataConstants=Inherit_from_model  RTWMemSecDataInternal=Inherit_from_model  RTWMemSecDataParameters=Inherit_from_model
      link override Model/ON Delay/Edge Detector/Model: RTWMemSecFuncInitTerm=Inherit_from_model  RTWMemSecFuncExecute=Inherit_from_model  RTWMemSecDataConstants=Inherit_from_model  RTWMemSecDataInternal=Inherit_from_model  RTWMemSecDataParameters=Inherit_from_model
      link override Model/ON Delay/Edge_Detector: RTWMemSecFuncInitTerm=Inherit_from_model  RTWMemSecFuncExecute=Inherit_from_model  RTWMemSecDataConstants=Inherit_from_model  RTWMemSecDataInternal=Inherit_from_model  RTWMemSecDataParameters=Inherit_from_model
      link override Model/ON Delay/Sample_and_Hold: RTWMemSecFuncInitTerm=Inherit_from_model  RTWMemSecFuncExecute=Inherit_from_model  RTWMemSecDataConstants=Inherit_from_model  RTWMemSecDataInternal=Inherit_from_model  RTWMemSecDataParameters=Inherit_from_model
      link override Model/ON Delay/Sample_and_Hold/Model: RTWMemSecFuncInitTerm=Inherit_from_model  RTWMemSecFuncExecute=Inherit_from_model  RTWMemSecDataConstants=Inherit_from_model  RTWMemSecDataInternal=Inherit_from_model  RTWMemSecDataParameters=Inherit_from_model
  Square2 : Math  Operator=square
  Switch : Switch  Criteria=u2 > Threshold  SaturateOnIntegerOverflow=off  InputSameDT=off
  _ : RelationalOperator  Operator=>  OutDataTypeStr=boolean  RndMeth=Simplest  InputSameDT=off
  AEB_STATUS : Outport
  INITIAL_SPEED : Outport  Port=2
  DISTANCE_TO_AVOID_COLLISION : Outport  Port=3
  wires:
  CAL.KM/Hr_TO_M/Hr_and_DISTANCE_TO_AVOID_COLLISION/2(DISTANCE_TO_AVOID_COLLISION) -> DISTANCE_TO_AVOID_COLLISION/1, Divide2/2  "DISTANCE_TO_AVOID_COLLISION"
  CAL.KM/Hr_TO_M/Hr_and_DISTANCE_TO_AVOID_COLLISION/1(INITIAL_SPEED_M/S) -> INITIAL_SPEED/1, Square2/1  "INITIAL_SPEED_M/S"
  BRAKING_DECCELERATION_APPLIED_BY_THE_DRIVER/1 -> _/1  "BRAKING_DECCELERATION_APPLIED_BY_THE_DRIVER"
  Multiply/1 -> _/2  "PARTIAL_BRAKING_DECCELERATION"
  Square2/1 -> Product3/3
  Constant4/1 -> Product3/1
  REACTION_TIME/1 -> Switch/1  "REACTION_TIME"
  SPEED_OF_EGO_VEHICLE/1 -> CAL.KM/Hr_TO_M/Hr_and_DISTANCE_TO_AVOID_COLLISION/1(INITIAL_SPEED)  "INITIAL_SPEED"
  Divide2/1 -> Divide3/2  "REQ_BRAKE_FORCE"
  _/1 -> REACTION_TIME/1  "COMPARING_THE_BOTH_BRAKING_DECCELERATION_VALUES"
  Constant5/1 -> Divide3/1, Product3/2  "MASS_OF_THE_VEHICLE"
  Product3/1 -> Divide2/1
  Constant1/1 -> Switch/3
  CAL_TTC/1 -> Compare_To_Constant/1
  Compare_To_Constant/1 -> Switch/2
  Switch/1 -> AEB_STATUS/1  "AEB_STATUS"
  Divide3/1 -> Multiply/1
  DISTANCE/1 -> CAL.KM/Hr_TO_M/Hr_and_DISTANCE_TO_AVOID_COLLISION/2(DISTANCE)  "DISTANCE"

== system AEB_MODEL_F/AEB/AEB_SYSTEM/CAL_TTC/condt_TIME_PHASE_PARITAL_BRAKING/REACTION_TIME ==
  In1 : Inport
  Enable : EnablePort
  Out1 : Outport
  wires:
  In1/1 -> Out1/1

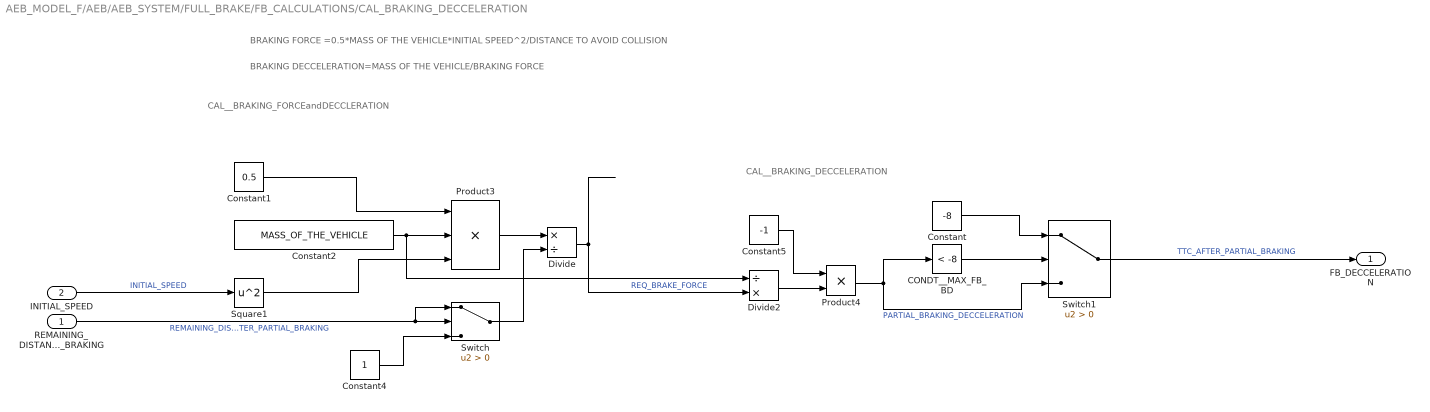
== system AEB_MODEL_F/AEB/AEB_SYSTEM/FULL_BRAKE/FB_CALCULATIONS/CAL_BRAKING_DECCELERATION ==
  note: CAL__BRAKING_DECCELERATION
  note: CAL__BRAKING_FORCEandDECCLERATION
  note: BRAKING FORCE =0.5*MASS OF THE VEHICLE*INITIAL SPEED^2/DISTANCE TO AVOID COLLISION
  note: BRAKING DECCELERATION=MASS OF THE VEHICLE/BRAKING FORCE
  REMAINING_DISTANCE_AFTER_PARTIAL_BRAKING : Inport
  INITIAL_SPEED : Inport  Port=2
  CONDT__MAX_FB_BD : simulink/Logic and Bit Operations/Compare To Constant  relop=<  const=-8  OutDataTypeStr=boolean
      settings: RTWMemSecFuncInitTerm=Inherit_from_model  RTWMemSecFuncExecute=Inherit_from_model  RTWMemSecDataConstants=Inherit_from_model  RTWMemSecDataInternal=Inherit_from_model  RTWMemSecDataParameters=Inherit_from_model
  Constant : Constant  Value=-8
  Constant1 : Constant  Value=0.5
  Constant2 : Constant  Value=MASS_OF_THE_VEHICLE
  Constant4 : Constant
  Constant5 : Constant  Value=-1
  Divide : Product  Inputs=*/
  Divide2 : Product  Inputs=/*
  Product3 : Product  Inputs=3
  Product4 : Product
  Square1 : Math  Operator=square
  Switch : Switch  Criteria=u2 > Threshold  SaturateOnIntegerOverflow=off  InputSameDT=off
  Switch1 : Switch  Criteria=u2 > Threshold  SaturateOnIntegerOverflow=off  InputSameDT=off
  FB_DECCELERATION : Outport
  wires:
  REMAINING_DISTANCE_AFTER_PARTIAL_BRAKING/1 -> Switch/1, Switch/2  "REMAINING_DISTANCE_AFTER_PARTIAL_BRAKING"
  Divide2/1 -> Product4/2
  Constant2/1 -> Divide2/1, Product3/2
  Product4/1 -> Switch1/3, CONDT__MAX_FB_BD/1  "PARTIAL_BRAKING_DECCELERATION"
  Constant1/1 -> Product3/1
  Divide/1 -> Divide2/2  "REQ_BRAKE_FORCE"
  Constant4/1 -> Switch/3
  Square1/1 -> Product3/3
  Product3/1 -> Divide/1
  Switch/1 -> Divide/2
  INITIAL_SPEED/1 -> Square1/1  "INITIAL_SPEED"
  Constant5/1 -> Product4/1
  Constant/1 -> Switch1/1
  Switch1/1 -> FB_DECCELERATION/1  "TTC_AFTER_PARTIAL_BRAKING"
  CONDT__MAX_FB_BD/1 -> Switch1/2

== system AEB_MODEL_F/AEB/AEB_SYSTEM/FULL_BRAKE/FB_CALCULATIONS/CAL_TTC ==
  INITIAL_SPEED_M/S : Inport
  SPEED_AFTER_FB_DECCELERATION : Inport  Port=2
  Constant6 : Constant
  Divide1 : Product  Inputs=/*
  Switch2 : Switch  Criteria=u2 > Threshold  SaturateOnIntegerOverflow=off  InputSameDT=off
  TTC_FOR_FULL_BRAKING : Outport
  wires:
  Constant6/1 -> Switch2/3
  Switch2/1 -> Divide1/1
  INITIAL_SPEED_M/S/1 -> Switch2/2, Switch2/1  "INITIAL_SPEED_M/S"
  SPEED_AFTER_FB_DECCELERATION/1 -> Divide1/2  "SPEED_AFTER_FB_DECCELERATION"
  Divide1/1 -> TTC_FOR_FULL_BRAKING/1

== system AEB_MODEL_F/AEB/AEB_SYSTEM/FULL_BRAKE/FB_CALCULATIONS/CAL_inital_after_decceleration_speed ==
  note: Speed after deceleration:
      | V = u + at
  INITIAL_SPEED : Inport
  TTC_FOR_FULL_BRAKING : Inport  Port=2
  FULL_BRAKING_DECCELERATION : Inport  Port=3
  Product5 : Product
  Subtract1 : Sum
  INITIAL_SPEED_M/S : Outport
  SPEED_AFTER_FB_DECCELERATION : Outport  Port=2
  wires:
  INITIAL_SPEED/1 -> Subtract1/1
  FULL_BRAKING_DECCELERATION/1 -> Product5/1  "FULL_BRAKING_DECCELERATION"
  Product5/1 -> Subtract1/2
  Subtract1/1 -> INITIAL_SPEED_M/S/1, SPEED_AFTER_FB_DECCELERATION/1  "INITIAL_SPEED_M/S"
  TTC_FOR_FULL_BRAKING/1 -> Product5/2  "TTC_FOR_FULL_BRAKING"

== system AEB_MODEL_F/AEB/AEB_SYSTEM/FULL_BRAKE/FB_CALCULATIONS/CAL_remainig_distance ==
  note: Remaining distance= ut + 1/2(at^2)
  INITIAL_SPEED : Inport
  REMAINING_DISTANCE_AFTER_PARTIAL_BRAKING : Inport  Port=2
  TTC_FOR_FULL_BRAKING : Inport  Port=3
  FB_DECCELERATION : Inport  Port=4
  Add1 : Sum
  Constant3 : Constant  Value=0.5
  Product1 : Product  Inputs=3
  Product2 : Product
  Square2 : Math  Operator=square
  Subtract3 : Sum  Inputs=+-
  remainig_distance : Outport
  wires:
  Add1/1 -> Subtract3/2
  TTC_FOR_FULL_BRAKING/1 -> Product2/2, Square2/1  "TTC_FOR_FULL_BRAKING"
  Square2/1 -> Product1/3
  Subtract3/1 -> remainig_distance/1  "remainig_distance"
  Product1/1 -> Add1/2
  Product2/1 -> Add1/1
  Constant3/1 -> Product1/1
  FB_DECCELERATION/1 -> Product1/2  "FB_DECCELERATION"
  REMAINING_DISTANCE_AFTER_PARTIAL_BRAKING/1 -> Subtract3/1  "REMAINING_DISTANCE_AFTER_PARTIAL_BRAKING"
  INITIAL_SPEED/1 -> Product2/1  "INITIAL_SPEED"
